simulink model "gm_test_switching_states_6Phase_without_delays"  (R2022a)
settings: Solver=FixedStepDiscrete  StartTime=0.0  StopTime=10.0  RelTol=1e-3
undefined symbols (not defined in the file or in its folder): f_c
settings Model: Creator=Andre Merx  LastModifiedBy=Andre Merx
settings SolverCC: AlgebraicLoopSolver=TrustRegion
settings DataIOCC: LimitDataPoints=on  SaveOutput=off  SaveTime=off
settings OptimizationCC: BlockReduction=off  ConditionallyExecuteInputs=off  DefaultParameterBehavior=Inlined  LifeSpan=inf
settings DebuggingCC: AlgebraicLoopMsg=error  InheritedTsInSrcMsg=none  SingleTaskRateTransMsg=error  UnconnectedInputMsg=warning  UnconnectedOutputMsg=warning  UnconnectedLineMsg=warning  AllowSymbolicDim=off  StrictBusMsg=ErrorOnBusTreatedAsVector  SFUnexpectedBacktrackingDiag=warning  SFNoUnconditionalDefaultTransitionDiag=warning  SFExecutionAtInitializationDiag=none  SFMachineParentedDataDiag=warning  ArithmeticOperatorsInVariantConditions=warning
settings HardwareCC: ProdBitPerPointer=32  ProdBitPerSizeT=32  ProdBitPerPtrDiffT=32  ProdLargestAtomicFloat=None  ProdIntDivRoundTo=Undefined  ProdEndianess=Unspecified  ProdWordSize=32  ProdHWDeviceType=ASIC/FPGA->ASIC/FPGA  ProdEqTarget=off
settings SFSimCC: SimUseLocalCustomCode=off  CustomCodeUndefinedFunction=UseInterfaceOnly
settings RTWCC: RTWUseLocalCustomCode=off
settings CodeAppCC: StateflowObjectComments=on
settings GRTTargetCC: TargetLangStandard=C89/C90 (ANSI)
settings ConfigComp: CovScope=ReferencedModels  CovMetricSettings=dw  CovSaveCumulativeToWorkspaceVar=on  CovSaveSingleToWorkspaceVar=on  CovExternalEMLEnable=off  CovSFcnEnable=off

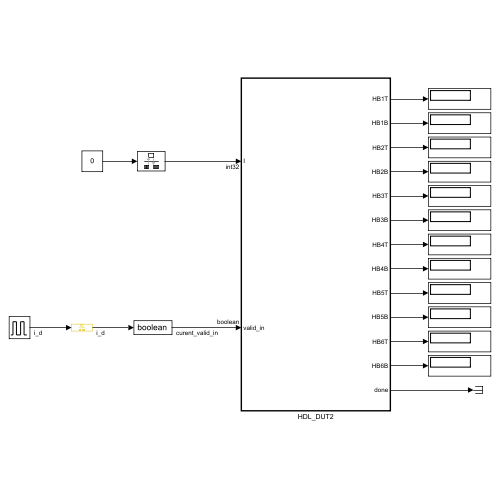
[thumbnail: Simulink's stored preview of the top-level diagram]
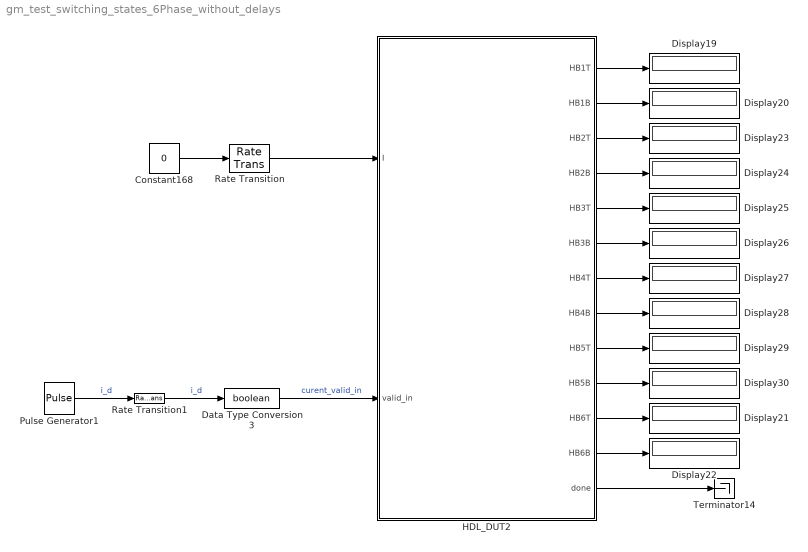
== system gm_test_switching_states_6Phase_without_delays ==
  Constant168 : Constant  Value=0  OutDataTypeStr=int32  SampleTime=-1
  Data Type Conversion3 : DataTypeConversion  OutDataTypeStr=boolean  SaturateOnIntegerOverflow=off  RndMeth=Floor
  Display{19..30} (12 alike) : Display
  HDL_DUT2 : Subsystem  TreatAsAtomicUnit=on
  Pulse Generator1 : DiscretePulseGenerator  PulseType=Time based  Period=1/f_c
  Rate Transition : RateTransition  OutPortSampleTime=Rt
  Rate Transition1 : RateTransition  OutPortSampleTime=Rt
  Terminator14 : Terminator
  wires:
  Pulse Generator1/1 -> Rate Transition1/1  "i_d"
  Data Type Conversion3/1 -> HDL_DUT2/2(valid_in)  "curent_valid_in"
  Rate Transition1/1 -> Data Type Conversion3/1  "i_d"
  HDL_DUT2/10(HB5B) -> Display30/1
  Constant168/1 -> Rate Transition/1
  HDL_DUT2/1(HB1T) -> Display19/1
  HDL_DUT2/2(HB1B) -> Display20/1
  HDL_DUT2/5(HB3T) -> Display25/1
  HDL_DUT2/7(HB4T) -> Display27/1
  HDL_DUT2/9(HB5T) -> Display29/1
  HDL_DUT2/3(HB2T) -> Display23/1
  HDL_DUT2/4(HB2B) -> Display24/1
  HDL_DUT2/8(HB4B) -> Display28/1
  HDL_DUT2/11(HB6T) -> Display21/1
  HDL_DUT2/12(HB6B) -> Display22/1
  HDL_DUT2/6(HB3B) -> Display26/1
  Rate Transition/1 -> HDL_DUT2/1(I)
  HDL_DUT2/13(done) -> Terminator14/1

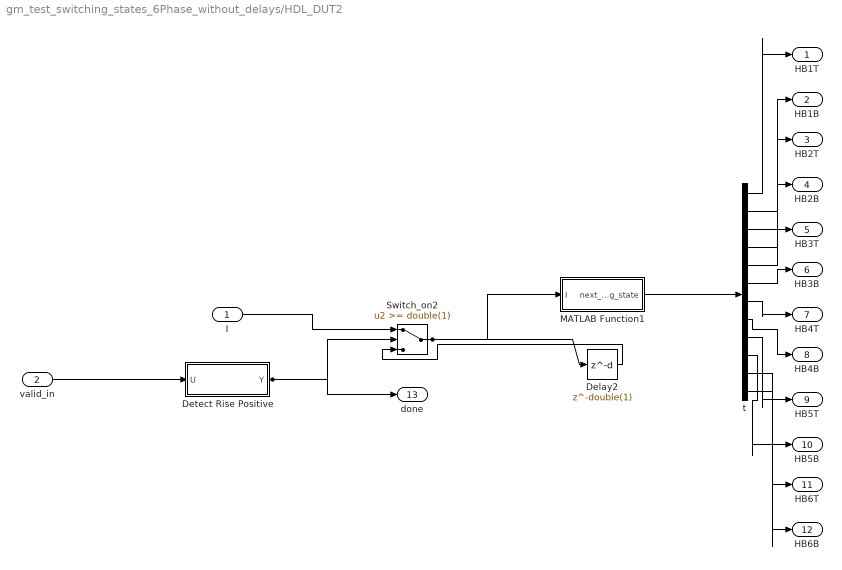
== system gm_test_switching_states_6Phase_without_delays/HDL_DUT2 ==
  I : Inport  OutDataTypeStr=int32  PortDimensions=1  SampleTime=1e-08
  valid_in : Inport  Port=2  OutDataTypeStr=boolean  PortDimensions=1  SampleTime=1e-08
  Delay2 : Delay  DelayLength=double(1)  InitialCondition=0  SampleTime=1e-08
  Detect Rise Positive : Subsystem  mask(Detect Rise Positive){vinit=double(0), InputProcessing=Elements as channels (sample based), OutDataTypeStr=boolean}
      mask prompts: vinit "Simulink:masks:InitialCondition_MP"; InputProcessing "Simulink:masks:InputProcessing_MP"; OutDataTypeStr "Simulink:masks:OutputDataType_MP"
      mask help: Simulink:masks:DetectRisePositive_MD
      mask init:
      | InputProcessing = 'Elements as channels (sample based)';
      | OutDataTypeStr = 'boolean';
      | vinit = double(0);
      mask TypeOptions InputProcessing: Simulink:masks:ColumnsAsChannelsFrameBased | Simulink:masks:ElementsAsChannelsSampleBased
      mask TypeOptions OutDataTypeStr: Simulink:masks:uint8 | Simulink:masks:boolean
      mask Display: fprintf('U > 0\n&  NOT\nU/z > 0')
  MATLAB Function1 : Subsystem
  Switch_on2 : Switch  Threshold=double(1)  OutDataTypeStr=int32  RndMeth=Simplest  SampleTime=1e-08  SaturateOnIntegerOverflow=off  InputSameDT=off
  t : Demux  Outputs=12
  HB1T : Outport  SampleTime=1e-08
  HB1B : Outport  Port=2  SampleTime=1e-08
  HB2T : Outport  Port=3  SampleTime=1e-08
  HB2B : Outport  Port=4  SampleTime=1e-08
  HB3T : Outport  Port=5  SampleTime=1e-08
  HB3B : Outport  Port=6  SampleTime=1e-08
  HB4T : Outport  Port=7  SampleTime=1e-08
  HB4B : Outport  Port=8  SampleTime=1e-08
  HB5T : Outport  Port=9  SampleTime=1e-08
  HB5B : Outport  Port=10  SampleTime=1e-08
  HB6T : Outport  Port=11  SampleTime=1e-08
  HB6B : Outport  Port=12  SampleTime=1e-08
  done : Outport  Port=13  SampleTime=1e-08
  wires:
  I/1 -> Switch_on2/1
  valid_in/1 -> Detect Rise Positive/1(U)
  Delay2/1 -> Switch_on2/3
  Detect Rise Positive/1(Y) -> Switch_on2/2, done/1
  MATLAB Function1/1(next_switching_state) -> t/1
  Switch_on2/1 -> Delay2/1, MATLAB Function1/1(I)
  t/1 -> HB1T/1
  t/2 -> HB1B/1
  t/3 -> HB2T/1
  t/4 -> HB2B/1
  t/5 -> HB3T/1
  t/6 -> HB3B/1
  t/7 -> HB4T/1
  t/8 -> HB4B/1
  t/9 -> HB5T/1
  t/10 -> HB5B/1
  t/11 -> HB6T/1
  t/12 -> HB6B/1

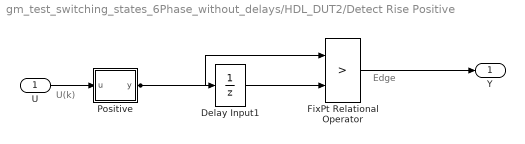
== system gm_test_switching_states_6Phase_without_delays/HDL_DUT2/Detect Rise Positive ==
  note: Edge
  note: U(k)
  U : Inport  OutDataTypeStr=boolean  SampleTime=1e-08
  Delay Input1 : UnitDelay  Description=Store in Global RAM  DisableCoverage=on  InitialCondition=vinit  SampleTime=-1  HasFrameUpgradeWarning=on
  FixPt Relational Operator : RelationalOperator  Operator=>  OutDataTypeStr=boolean  ZeroCross=off  InputSameDT=off
  Positive : Subsystem  mask(Compare To Zero){relop=>, OutDataTypeStr=boolean, ZeroCross=off}
      mask prompts: relop "Simulink:masks:Operator_MP"; OutDataTypeStr "Simulink:masks:OutputDataType_MP"; ZeroCross "Simulink:masks:EnableZerocrossingDetection_MP"
      mask help: Simulink:masks:CompareToZero_MD
      mask init:
      | OutDataTypeStr = 'boolean';
      | ZeroCross = 'off';
      | blkName = 'test_switching_states_6Phase_without_delays/HDL_DUT2/Detect Rise\nPositive/Positive';
      | relop = '>';
      | setValue = 'boolean';
      mask TypeOptions relop: == | ~= | < | <= | >= | >
      mask TypeOptions OutDataTypeStr: Simulink:masks:uint8 | Simulink:masks:boolean
      mask Callback ZeroCross: sl('zeroCrossEnable', gcbh);
      mask Display: disp([relop,' 0'])
  Y : Outport  SampleTime=1e-08
  wires:
  U/1 -> Positive/1(u)
  Delay Input1/1 -> FixPt Relational Operator/2
  FixPt Relational Operator/1 -> Y/1
  Positive/1(y) -> FixPt Relational Operator/1, Delay Input1/1

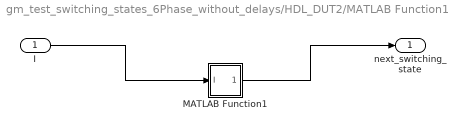
== system gm_test_switching_states_6Phase_without_delays/HDL_DUT2/MATLAB Function1 ==
  I : Inport  OutDataTypeStr=int32  PortDimensions=1  SampleTime=1e-08
  MATLAB Function1 : MATLAB Function  TreatAsAtomicUnit=on
  next_switching_state : Outport  SampleTime=1e-08  VectorParamsAs1DForOutWhenUnconnected=off
  wires:
  I/1 -> MATLAB Function1/1(I)
  MATLAB Function1/1(next_switching_state) -> next_switching_state/1

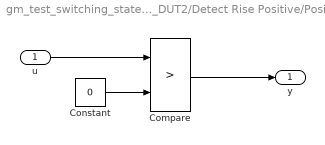
== system gm_test_switching_states_6Phase_without_delays/HDL_DUT2/Detect Rise Positive/Positive ==
  u : Inport  OutDataTypeStr=boolean  SampleTime=1e-08
  Compare : RelationalOperator  Operator=>  OutDataTypeStr=boolean  ZeroCross=off
  Constant : Constant  DisableCoverage=on  Value=0  OutDataTypeStr=Inherit: Inherit via back propagation  SampleTime=-1  PreserveConstantTs=on
  y : Outport  SampleTime=1e-08
  wires:
  u/1 -> Compare/1
  Compare/1 -> y/1
  Constant/1 -> Compare/2

== matlab function gm_test_switching_states_6Phase_without_delays/HDL_DUT2/MATLAB Function1/MATLAB Function1 ==
  data: I input; next_switching_state output
function next_switching_state = fcn(I)

    % Possible switching states of the 6-Phase 2-level inverter
    possible_swichting_states = [0	1	0	1	0	1	0	1	0	1	0	1;
                                1	0	0	1	0	1	0	1	0	1	0	1;
                                0	1	1	0	0	1	0	1	0	1	0	1;
                                1	0	1	0	0	1	0	1	0	1	0	1;
                                0	1	0	1	1	0	0	1	0	1	0	1;
                                1	0	0	1	1	0	0	1	0	1	0	1;
                                0	1	1	0	1	0	0	1	0	1	0	1;
                                1	0	1	0	1	0	0	1	0	1	0	1;
                                0	1	0	1	0	1	1	0	0	1	0	1;
                                1	0	0	1	0	1	1	0	0	1	0	1;
                                0	1	1	0	0	1	1	0	0	1	0	1;
                                1	0	1	0	0	1	1	0	0	1	0	1;
                                0	1	0	1	1	0	1	0	0	1	0	1;
                                1	0	0	1	1	0	1	0	0	1	0	1;
                                0	1	1	0	1	0	1	0	0	1	0	1;
                                1	0	1	0	1	0	1	0	0	1	0	1;
                                0	1	0	1	0	1	0	1	1	0	0	1;
                                1	0	0	1	0	1	0	1	1	0	0	1;
                                0	1	1	0	0	1	0	1	1	0	0	1;
                                1	0	1	0	0	1	0	1	1	0	0	1;
                                0	1	0	1	1	0	0	1	1	0	0	1;
                                1	0	0	1	1	0	0	1	1	0	0	1;
                                0	1	1	0	1	0	0	1	1	0	0	1;
                                1	0	1	0	1	0	0	1	1	0	0	1;
                                0	1	0	1	0	1	1	0	1	0	0	1;
                                1	0	0	1	0	1	1	0	1	0	0	1;
                                0	1	1	0	0	1	1	0	1	0	0	1;
                                1	0	1	0	0	1	1	0	1	0	0	1;
                                0	1	0	1	1	0	1	0	1	0	0	1;
                                1	0	0	1	1	0	1	0	1	0	0	1;
                                0	1	1	0	1	0	1	0	1	0	0	1;
                                1	0	1	0	1	0	1	0	1	0	0	1;
                                0	1	0	1	0	1	0	1	0	1	1	0;
                                1	0	0	1	0	1	0	1	0	1	1	0;
                                0	1	1	0	0	1	0	1	0	1	1	0;
                                1	0	1	0	0	1	0	1	0	1	1	0;
                                0	1	0	1	1	0	0	1	0	1	1	0;
                                1	0	0	1	1	0	0	1	0	1	1	0;
                                0	1	1	0	1	0	0	1	0	1	1	0;
                                1	0	1	0	1	0	0	1	0	1	1	0;
                                0	1	0	1	0	1	1	0	0	1	1	0;
                                1	0	0	1	0	1	1	0	0	1	1	0;
                                0	1	1	0	0	1	1	0	0	1	1	0;
                                1	0	1	0	0	1	1	0	0	1	1	0;
                                0	1	0	1	1	0	1	0	0	1	1	0;
                                1	0	0	1	1	0	1	0	0	1	1	0;
                                0	1	1	0	1	0	1	0	0	1	1	0;
                                1	0	1	0	1	0	1	0	0	1	1	0;
                                0	1	0	1	0	1	0	1	1	0	1	0;
                                1	0	0	1	0	1	0	1	1	0	1	0;
                                0	1	1	0	0	1	0	1	1	0	1	0;
                                1	0	1	0	0	1	0	1	1	0	1	0;
                                0	1	0	1	1	0	0	1	1	0	1	0;
                                1	0	0	1	1	0	0	1	1	0	1	0;
                                0	1	1	0	1	0	0	1	1	0	1	0;
                                1	0	1	0	1	0	0	1	1	0	1	0;
                                0	1	0	1	0	1	1	0	1	0	1	0;
                                1	0	0	1	0	1	1	0	1	0	1	0;
                                0	1	1	0	0	1	1	0	1	0	1	0;
                                1	0	1	0	0	1	1	0	1	0	1	0;
                                0	1	0	1	1	0	1	0	1	0	1	0;
                                1	0	0	1	1	0	1	0	1	0	1	0;
                                0	1	1	0	1	0	1	0	1	0	1	0;
                                1	0	1	0	1	0	1	0	1	0	1	0];

    % Initial condition
    if I==0
        I=int32(1);
    end

    % Output switching state
    next_switching_state=boolean(possible_swichting_states(I,:))';

end
